simulink model "Thermofluids_LV"  (R2025a)
settings: Solver=VariableStepAuto  StartTime=0.0  StopTime=10.0  RelTol=1e-3
settings Model: Creator=mu22504  LastModifiedBy=Adam

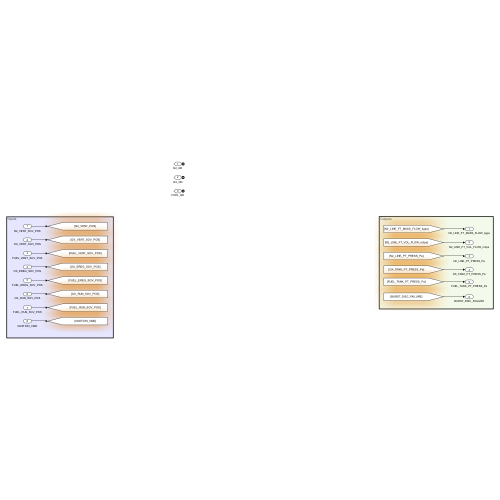
[thumbnail: Simulink's stored preview of the top-level diagram]
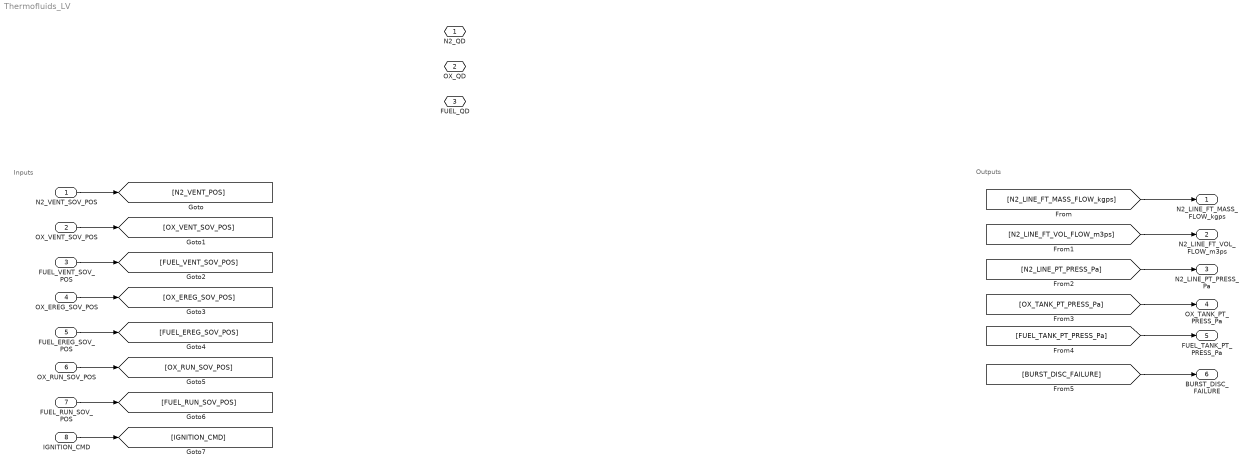
== system Thermofluids_LV ==
  note: Inputs
  note: Outputs
  N2_VENT_SOV_POS : Inport
  OX_VENT_SOV_POS : Inport  Port=2
  FUEL_VENT_SOV_POS : Inport  Port=3
  OX_EREG_SOV_POS : Inport  Port=4
  FUEL_EREG_SOV_POS : Inport  Port=5
  OX_RUN_SOV_POS : Inport  Port=6
  FUEL_RUN_SOV_POS : Inport  Port=7
  IGNITION_CMD : Inport  Port=8
  N2_QD : PMIOPort  Side=Left
  OX_QD : PMIOPort  Port=2  Side=Left
  FUEL_QD : PMIOPort  Port=3  Side=Left
  N2_LINE_FT_MASS_FLOW_kgps : Outport
  N2_LINE_FT_VOL_FLOW_m3ps : Outport  Port=2
  N2_LINE_PT_PRESS_Pa : Outport  Port=3
  OX_TANK_PT_PRESS_Pa : Outport  Port=4
  FUEL_TANK_PT_PRESS_Pa : Outport  Port=5
  BURST_DISC_FAILURE : Outport  Port=6
  wires:
  N2_VENT_SOV_POS/1 -> [N2_VENT_POS]
  [N2_LINE_FT_MASS_FLOW_kgps] -> N2_LINE_FT_MASS_FLOW_kgps/1
  OX_VENT_SOV_POS/1 -> [OX_VENT_SOV_POS]
  FUEL_VENT_SOV_POS/1 -> [FUEL_VENT_SOV_POS]
  OX_EREG_SOV_POS/1 -> [OX_EREG_SOV_POS]
  FUEL_EREG_SOV_POS/1 -> [FUEL_EREG_SOV_POS]
  OX_RUN_SOV_POS/1 -> [OX_RUN_SOV_POS]
  FUEL_RUN_SOV_POS/1 -> [FUEL_RUN_SOV_POS]
  [N2_LINE_FT_VOL_FLOW_m3ps] -> N2_LINE_FT_VOL_FLOW_m3ps/1
  [N2_LINE_PT_PRESS_Pa] -> N2_LINE_PT_PRESS_Pa/1
  [OX_TANK_PT_PRESS_Pa] -> OX_TANK_PT_PRESS_Pa/1
  [FUEL_TANK_PT_PRESS_Pa] -> FUEL_TANK_PT_PRESS_Pa/1
  [BURST_DISC_FAILURE] -> BURST_DISC_FAILURE/1
  IGNITION_CMD/1 -> [IGNITION_CMD]
